simulink model "sf_tetris2"  (Simulink 7.6)
settings: Solver=FixedStepDiscrete  StartTime=0.0  StopTime=inf  FixedStep=1  RelTol=1e-3
libraries: simulink x1
CloseFcn:
  | sf_tetris2_gui('close');
settings Model: Creator=The MathWorks Inc.  ExtModeAutoUpdateStatusClock=off
settings OptimizationCC: InitFltsAndDblsToZero=on  EfficientMapNaN2IntZero=off
settings DebuggingCC: SaveWithParameterizedLinksMsg=none  SignalResolutionControl=TryResolveAllWithWarning  StrictBusMsg=Warning
settings SFSimCC: SFSimEnableDebug=off  SFSimOverflowDetection=off  SFSimEcho=off  SimParseCustomCode=off
settings GRTTargetCC: TargetFcnLib=ansi_tfl_tmw.mat

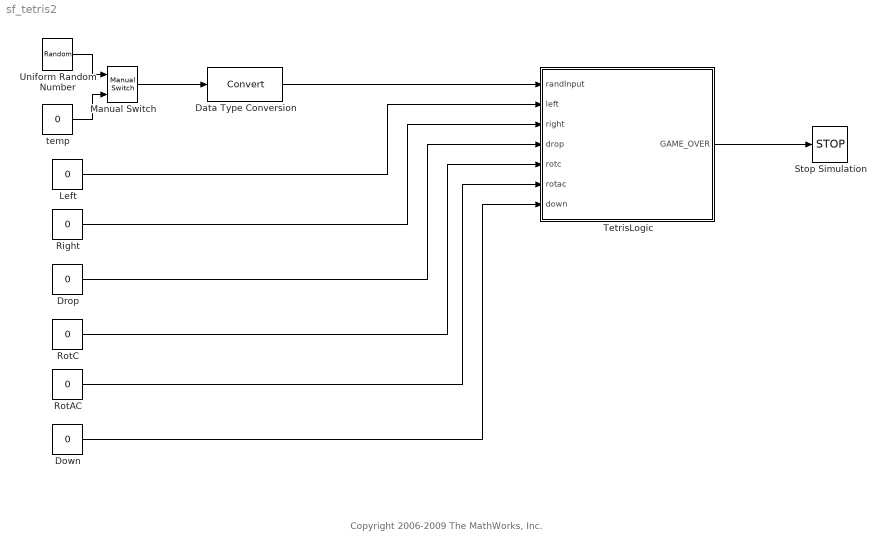
== system sf_tetris2 ==
  note: Copyright 2006-2009 The MathWorks, Inc.
  Data Type Conversion : DataTypeConversion
  Down : Constant  Value=0
  Drop : Constant  Value=0
  Left : Constant  Value=0  OutDataTypeStr=double
  Manual Switch : simulink/Signal Routing/Manual Switch  SystemSampleTime=-1  sw=1  action=0  varsize=off
  Right : Constant  Value=0
  RotAC : Constant  Value=0
  RotC : Constant  Value=0
  Stop Simulation : Stop
  TetrisLogic : Stateflow chart  TreatAsAtomicUnit=on
  Uniform Random Number : UniformRandomNumber  Minimum=0  Maximum=7  Seed=20  SampleTime=0
  temp : Constant  Value=0
  wires:
  Data Type Conversion/1 -> TetrisLogic/1(randInput)
  Uniform Random Number/1 -> Manual Switch/1
  temp/1 -> Manual Switch/2
  Manual Switch/1 -> Data Type Conversion/1
  Left/1 -> TetrisLogic/2(left)
  Right/1 -> TetrisLogic/3(right)
  Drop/1 -> TetrisLogic/4(drop)
  RotC/1 -> TetrisLogic/5(rotc)
  RotAC/1 -> TetrisLogic/6(rotac)
  Down/1 -> TetrisLogic/7(down)
  TetrisLogic/1(GAME_OVER) -> Stop Simulation/1

== stateflow chart TetrisLogic ==
  state MainArea [parallel]
    settings: executionOrder=2
    state Stopped
    state GameOver
      en:
      send(GAME_OVER);
    state NewShape
      en:
      shape = WaitingArea.shape;
      py = ARENA_HEIGHT;
      px = ARENA_WIDTH/2 + 1;
      send(WaitingArea.NEW);
    state move(dx, dy) [function]
      (default) -> (junction 43) : [!isTouching(px+dx,py+dy)]
          | {
          | px += dx;
          | py += dy;
          | }
    state initArena [function]
      note: Make the "walls" for the arena
      (default) -> (junction 61) : {arena = 0;
          | i = 0;}
      (junction 61) -> (junction 62) [order 1] : [i < ARENA_HEIGHT+1]
      (junction 61) -> (junction 64) [order 2] : {i = 0;}
      (junction 62) -> (junction 63) : {
          | arena[i][0] = 1;
          | arena[i][ARENA_WIDTH+1] = 1;
          | }
      (junction 63) -> (junction 61) : {i++;}
      (junction 65) -> (junction 53) : {
          | arena[0][i] = 1;
          | }
      (junction 64) -> (junction 65) [order 1] : [i < ARENA_WIDTH+2]
      (junction 64) -> (junction 47) [order 2]
      (junction 53) -> (junction 64) : {i++;}
    state ist = isTouching(x,y) [function]
      (junction 46) -> (junction 44) [order 1] : [y+i >= 0 && y+i < ARENA_HEIGHT+1 ...
          |  && x+j >= 0 && x+j < ARENA_WIDTH+2]
      (junction 71) -> (junction 45) [order 2] : {ist=0;}
      (junction 44) -> (junction 49) : [shape[i][j] && arena[y+i][x+j]]
          | {
          | ist = 1;
          | }
      (junction 48) -> (junction 71) [order 2] : {i++;}
      (junction 46) -> (junction 48) [order 2] : {j++;}
      (junction 71) -> (junction 48) [order 1] : [i<4]{j=0;}
      (junction 48) -> (junction 46) [order 1] : [j<4]
      (default) -> (junction 71) : {i=0;}
    state FreezeShape
      en:
      freeze();
      shape = 0;
    state Score
      state Tetris
        en:
        // can do some animation
        // here
      state Done
        en:
        calcScore();
      state yesno = isRowMade(r) [function]
        (default) -> (junction 73) : {i = 0;}
        (junction 73) -> (junction 74) [order 1] : [i < ARENA_WIDTH]
        (junction 75) -> (junction 73) : {i++;}
        (junction 74) -> (junction 75) [order 2]
        (junction 74) -> (junction 76) [order 1] : [arena[r][i+1]==0]
            | {yesno = 0;}
        (junction 73) -> (junction 77) [order 2] : {yesno = 1;}
      state clearRow(r) [function]
        (junction 67) -> (junction 68) : {arena[i][j+1] = ...
            | arena[i+1][j+1];}
        (junction 66) -> (junction 70) [order 2]
        (junction 68) -> (junction 66) : {j++;}
        (junction 66) -> (junction 67) [order 1] : [j < ARENA_WIDTH]
        (junction 79) -> (junction 66) : {j=0;}
        (junction 78) -> (junction 69) [order 2]
        (default) -> (junction 78) : {i=r;}
        (junction 78) -> (junction 79) [order 1] : [i < ARENA_HEIGHT]
        (junction 70) -> (junction 78) : {i++;}
      state ClearCompletedRows
        state Delay
        state Clear
          en:
          clearRow(botRow);
          rowsCleared++;
          totalRowsCleared++;
        (default) -> Clear
        Clear -> Delay [order 1] : [isRowMade(botRow)]
        Delay -> Clear : [after(20,tick)]
      Clear -> Tetris [order 2] : [rowsCleared == 4]
      (junction 85) -> (junction 82) [order 1] : [botRow <= ARENA_HEIGHT]
      (default) -> (junction 81)
      (junction 82) -> (junction 85) [order 1] : [!isRowMade(botRow)]{botRow++;}
      (junction 85) -> Done [order 2] : //no row fully formed
      (junction 82) -> ClearCompletedRows [order 2] : // botRow is bottom most
          | // fully formed row
      Clear -> Done [order 3]
      Tetris -> Done : [after(10,tick)]
      (junction 81) -> (junction 85) : {
          | rowsCleared=0;
          | botRow = 1;
          | }
    state freeze [function]
      (junction 72) -> (junction 54) [order 1] : [j<4]
      (junction 52) -> (junction 51) [order 2]
      (junction 51) -> (junction 72) : {j++;}
      (junction 54) -> (junction 51) [order 2]
      (junction 50) -> (junction 55) [order 2]
      (junction 72) -> (junction 50) [order 2] : {i++;}
      (junction 52) -> (junction 51) [order 1] : [!arena[py+i][px+j] && shape[i][j]]
          | {arena[py+i][px+j] = shape[i][j];}
      (junction 54) -> (junction 52) [order 1] : [py+i >= 0 && py+i < ARENA_HEIGHT+1 ...
          |  && px+j >= 0 && px+j < ARENA_WIDTH+2]
      (default) -> (junction 50) : {
          | i=0;
          | }
      (junction 50) -> (junction 72) [order 1] : [i<4]{j=0;}
    state Moving
      state MoveFast
        MoveFast -> (junction 83) : {
            | move(0,-1);
            | dropHeight++;
            | }
      state MoveSlowly
        state DOWN [parallel]
          settings: executionOrder=5
          state Down
            en:
            move(0,-1);
          state Idle
            en: counter = 0;
            du: counter++;
          MainArea.Moving.MoveSlowly.DOWN.Idle -> Down : [after(15-3*level+3,tick)]
          Down -> MainArea.Moving.MoveSlowly.DOWN.Idle
          (default) -> Down
        state RIGHT [parallel]
          settings: executionOrder=1
          RIGHT -> (junction 87) : [hasChanged(right)]{move(1,0);}
        state ROTAC [parallel]
          settings: executionOrder=3
          ROTAC -> (junction 89) : [hasChanged(rotac)]{shape = rotateAC(shape);}
          (junction 89) -> (junction 90) : [isTouching(px,py)]{shape = rotateC(shape);}
        state LEFT [parallel]
          settings: executionOrder=2
          LEFT -> (junction 88) : [hasChanged(left)]{move(-1,0);}
        state ROTC [parallel]
          settings: executionOrder=4
          ROTC -> (junction 91) : [hasChanged(rotc)]{shape = rotateC(shape);}
          (junction 91) -> (junction 92) : [isTouching(px,py)]{shape = rotateAC(shape);}
        state DOWN_USER [parallel]
          settings: executionOrder=6
          DOWN_USER -> (junction 93) : [hasChanged(down)]{move(0,-1);}
      (default) -> MoveSlowly : {dropHeight=0;}
      MoveSlowly -> MoveFast : [hasChanged(drop)]
    state NextLevel [group]
      (junction 86) -> (junction 84) [order 2]
      (junction 80) -> (junction 84) : [level < 6]
          | {level++;}
      (junction 86) -> (junction 80) [order 1] : [totalRowsCleared >= 10]
          | {
          | totalRowsCleared = 0;
          | score += 1000*level;
          | initArena();
          | }
    Moving -> Stopped : [isTouching(px,py-1)]
    Stopped -> GameOver [order 1] : [py >= ARENA_HEIGHT]
    Done -> (junction 86)
    Stopped -> FreezeShape [order 2]
    NewShape -> Moving
    (default) -> NewShape : {initArena();}
    FreezeShape -> Score
    (junction 84) -> NewShape
  state Draw [parallel]
    en:
    ml.sf_tetris2_gui('init');
    du:
    ml.sf_tetris2_gui('draw', MainArea.arena, MainArea.shape, ...
    WaitingArea.shape, MainArea.px, MainArea.py, ...
    MainArea.score, MainArea.level, MainArea.totalRowsCleared);
    settings: executionOrder=3
  state WaitingArea [parallel]
    en:
    setShapes();
    settings: executionOrder=1
    state createShapeFrom(num) [function]
      (junction 57) -> (junction 60) [order 2]
      (default) -> (junction 57) : {i = 0;}
      (junction 57) -> (junction 58) [order 1] : [i < 16]
      (junction 58) -> (junction 59) : {
          | r = i/4;
          | c = i%%4;
          | b = (shapes[num] >> i) & 0x0001;
          | shape[r][c] = b*(num+2);
          | }
      (junction 59) -> (junction 57) : {i++;}
    state setShapes [function]
      (default) -> (junction 56) : {
          | shapes[0] = 0x00F0;
          | shapes[1] = 0x2260;
          | shapes[2] = 0x4460;
          | shapes[3] = 0x0660;
          | shapes[4] = 0x0360;
          | shapes[5] = 0x0C60;
          | shapes[6] = 0x0270;
          | }
    state Idle
      en:
      createShapeFrom(randInput);
    WaitingArea.Idle -> WaitingArea.Idle : NEW
  state newShape = rotateAC(shape) [function]
    (default) -> (junction 41) : {
        | newShape[0][0] = shape[3][0];
        | newShape[0][1] = shape[2][0];
        | newShape[0][2] = shape[1][0];
        | newShape[0][3] = shape[0][0];
        |
        | newShape[1][0] = shape[3][1];
        | newShape[1][1] = shape[2][1];
        | newShape[1][2] = shape[1][1];
        | newShape[1][3] = shape[0][1];
        |
        | newShape[2][0] = shape[3][2];
        | newShape[2][1] = shape[2][2];
        | newShape[2][2] = shape[1][2];
        | newShape[2][3] = shape[0][2];
        |
        | newShape[3][0] = shape[3][3];
        | newShape[3][1] = shape[2][3];
        | newShape[3][2] = shape[1][3];
        | newShape[3][3] = shape[0][3];
        | }
  state newShape = rotateC(shape) [function]
    (default) -> (junction 42) : {
        | newShape[0][0] = shape[0][3];
        | newShape[0][1] = shape[1][3];
        | newShape[0][2] = shape[2][3];
        | newShape[0][3] = shape[3][3];
        |
        | newShape[1][0] = shape[0][2];
        | newShape[1][1] = shape[1][2];
        | newShape[1][2] = shape[2][2];
        | newShape[1][3] = shape[3][2];
        |
        | newShape[2][0] = shape[0][1];
        | newShape[2][1] = shape[1][1];
        | newShape[2][2] = shape[2][1];
        | newShape[2][3] = shape[3][1];
        |
        | newShape[3][0] = shape[0][0];
        | newShape[3][1] = shape[1][0];
        | newShape[3][2] = shape[2][0];
        | newShape[3][3] = shape[3][0];
        | }
  data: arena local uint8 size=[ARENA_HEIGHT+1, ARENA_WIDTH+2]; px local int8; py local int8; dropHeight local double; shape local uint8 size=[4,4]; level local uint8 =1; totalRowsCleared local int32; score local double; num function_input uint16; r temporary uint8; c temporary uint8; b temporary uint8; i temporary uint8; shapes local uint16 size=7; shape local uint8 size=[4,4]; dx function_input int8; dy function_input int8; shape function_input uint8 size=[4,4]; newShape function_output uint8 size=[4,4]; shape function_input uint8 size=[4,4]; newShape function_output uint8 size=[4,4]; i temporary uint8; x function_input int8; y function_input int8; ist function_output int8; i temporary int8; j temporary int8; rowsCleared local int8; botRow local int8; i temporary int8; j temporary int8; yesno function_output double; i temporary int8; r function_input int8; i temporary int8; j temporary int8; r function_input double; counter local double; randInput input double; left input double; right input double; drop input double; rotc input double; rotac input double; down input double
  events: NEW local EITHER_EDGE_EVENT; GAME_OVER output EITHER_EDGE_EVENT
  function calcScore:
    | function calcScore
    | % increments the score according to the number of rows currently cleared
    | 
    | persistent linesToScoreMap
    | if isempty(linesToScoreMap)
    |     linesToScoreMap = [40, 100, 300, 1200];
    | end
    | 
    | if rowsCleared > 0
    |     score = score + double(linesToScoreMap(rowsCleared)*level);
    | end
    | score = score + double(dropHeight*level*10);
